simulink model "simTP2_2020a"  (R2020a)
settings: Solver=ode4  StartTime=0.0  StopTime=10  FixedStep=1e-5  RelTol=1e-7
values from neighbouring files (symbols this model uses):
  dy0 = 0    [scriptTP2.m]
  g = 9.8    [scriptTP2.m]
  K = 0.0005    [scriptTP2.m]
  m = 0.1    [scriptTP2.m]
  y0 = 0.01    [scriptTP2.m]
libraries: simulink x1
settings Model: Creator=yariba  LastModifiedBy=yariba
settings DebuggingCC: UnconnectedInputMsg=none  UnconnectedOutputMsg=none  UnconnectedLineMsg=none

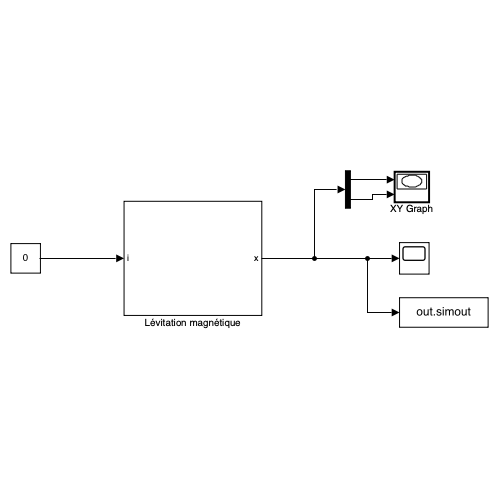
[thumbnail: Simulink's stored preview of the top-level diagram]
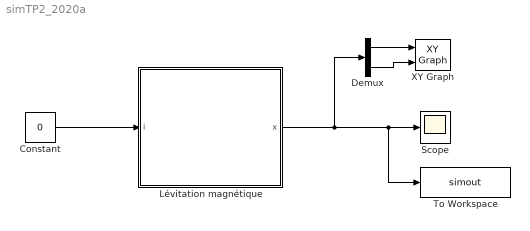
== system simTP2_2020a ==
  Constant : Constant  Value=0
  Demux : Demux  Outputs=2
  Lévitation magnétique : Subsystem
  Scope : Scope
  To Workspace : ToWorkspace  VariableName=simout  SaveFormat=Timeseries  SampleTime=-1
  XY Graph : simulink/Sinks/XY Graph  xmin=-1  xmax=1  ymin=-1  ymax=1  st=-1
  wires:
  Lévitation magnétique/1(x) -> Demux/1, To Workspace/1, Scope/1
  Demux/1 -> XY Graph/1
  Demux/2 -> XY Graph/2
  Constant/1 -> Lévitation magnétique/1(i)

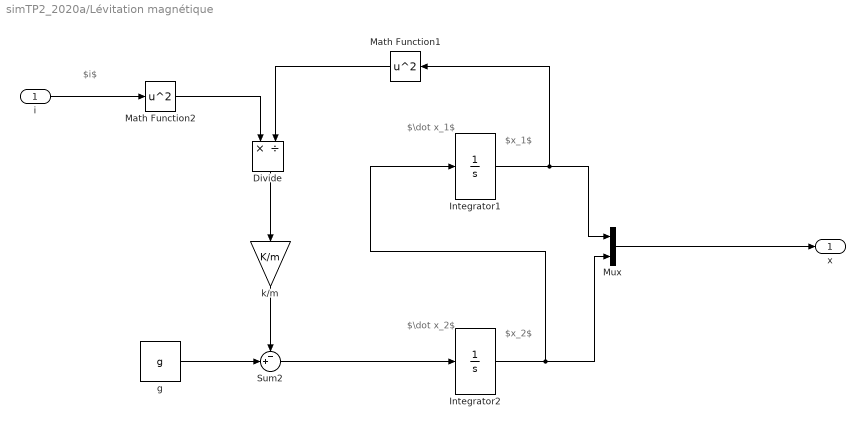
== system simTP2_2020a/Lévitation magnétique ==
  note: $x_1$
  note: $x_2$
  note: $\dot x_1$
  note: $\dot x_2$
  note: $i$
  i : Inport
  Divide : Product  Inputs=*/
  Integrator1 : Integrator  InitialCondition=y0
  Integrator2 : Integrator  InitialCondition=dy0
  Math Function1 : Math  Operator=square  SaturateOnIntegerOverflow=on
  Math Function2 : Math  Operator=square  SaturateOnIntegerOverflow=on
  Mux : Mux  Inputs=2
  Sum2 : Sum  Inputs=-+|
  g : Constant  Value=g
  k/m : Gain  Gain=K/m
  x : Outport
  wires:
  Integrator2/1 -> Integrator1/1, Mux/2
  Divide/1 -> k/m/1
  Mux/1 -> x/1
  Integrator1/1 -> Math Function1/1, Mux/1
  k/m/1 -> Sum2/1
  Sum2/1 -> Integrator2/1
  g/1 -> Sum2/2
  i/1 -> Math Function2/1
  Math Function1/1 -> Divide/2
  Math Function2/1 -> Divide/1
